simulink model "case_study_1"  (R2022a)
settings: Solver=VariableStepAuto  StartTime=0.0  StopTime=100  RelTol=1e-3
settings Model: Creator=spinolam  LastModifiedBy=spinolam

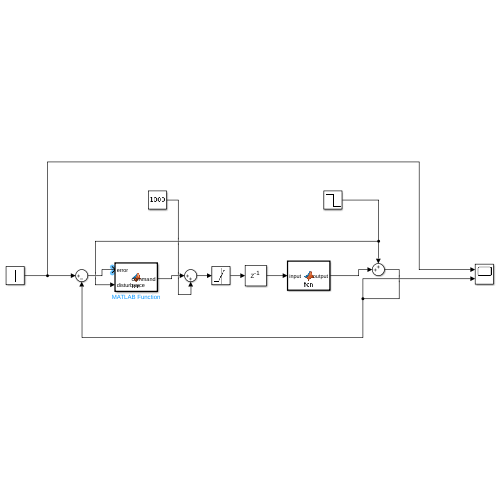
[thumbnail: Simulink's stored preview of the top-level diagram]
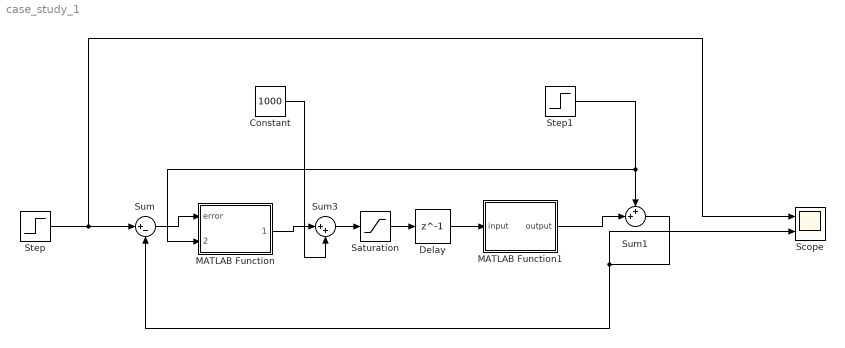
== system case_study_1 ==
  Constant : Constant  Value=1000
  Delay : Delay  DelayLength=1  InitialCondition=1000  SampleTime=1
  MATLAB Function : MATLAB Function  TreatAsAtomicUnit=on
  MATLAB Function1 : MATLAB Function  TreatAsAtomicUnit=on
  Saturation : Saturate  UpperLimit=inf  LowerLimit=1000
  Scope : Scope  NumInputPorts=2
  Step : Step  Time=20  Before=1000  After=1100
  Step1 : Step  Time=50  After=-100
  Sum : Sum  Inputs=|+-
  Sum1 : Sum  Inputs=++|
  Sum3 : Sum  Inputs=|++
  wires:
  Step/1 -> Scope/1, Sum/1
  Sum/1 -> MATLAB Function/1(error)
  MATLAB Function1/1(output) -> Sum1/2
  Sum1/1 -> Scope/2, Sum/2
  MATLAB Function/1(command) -> Sum3/1
  Sum3/1 -> Saturation/1
  Constant/1 -> Sum3/2
  Saturation/1 -> Delay/1
  Delay/1 -> MATLAB Function1/1(input)
  Step1/1 -> MATLAB Function/2(disturbance), Sum1/1

== matlab function case_study_1/MATLAB Function ==
  data: error input; command output; disturbance input
function command = fcn(error,disturbance)
persistent z disturbance_old
kp=0.3; ki=0.3; kf=-0.5;
if isempty(z)s
    z=0;
    disturbance_old=0;
end


z=z+error;
command= ki*z + kp*error +kf*disturbance_old -kf*disturbance;
disturbance_old = disturbance;

== matlab function case_study_1/MATLAB Function1 ==
  data: input input; output output
function output = fcn(input)
persistent output_old
alpha=0.5;
if isempty(output_old)
    output_old=1000;
end


output_new= (1-alpha)*output_old + alpha*input ;
output= output_old;
output_old=output_new;
